simulink model "krzywdalab_tf_si"  (R2023b)
settings: Solver=VariableStepAuto  StartTime=0.0  StopTime=10.0  RelTol=1e-3
values from neighbouring files (symbols this model uses):
  fwe10 = tab_fwe1(it)    [krzywdalab8.m]
  fwe20 = 0.1 * fwe2max    [krzywdalab8.m]
  h10 = (fwe10 + a1 * h20) / a1    [krzywdalab8.m]
  h20 = (fwe10 + fwe20) / a2    [krzywdalab8.m]
  M = [(A1 * A2) (a_1 * A1 + a_2 * A1 + a_1 * A2) a_1*a_2]    [feedback_cascade_transfer_function.m]    (also in krzywdalab8.m = [(A1*A2) (a1*A1+a2*A1+a1*A2) a1*a2])
  N_11 = [A2 (a_1 + a_2)]    [feedback_cascade_transfer_function.m]    (also in krzywdalab8.m = [A2 (a1+a2)])
  N_21 = [a_1]    [feedback_cascade_transfer_function.m]    (also in krzywdalab8.m = [a1])
  N_22 = [A1 a_1]    [feedback_cascade_transfer_function.m]    (also in krzywdalab8.m = [A1 a1])
  T0 = 2    [feedback_cascade_state.m]    (also in feedback_cascade_transfer_function.m; krzywdalab8.m)
settings Model: Creator=igorkrzywda  LastModifiedBy=igorkrzywda

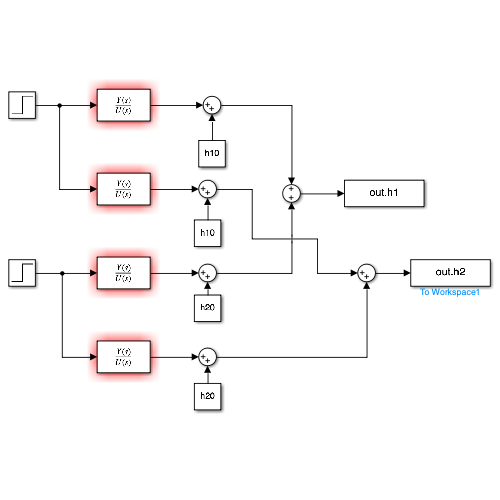
[thumbnail: Simulink's stored preview of the top-level diagram]
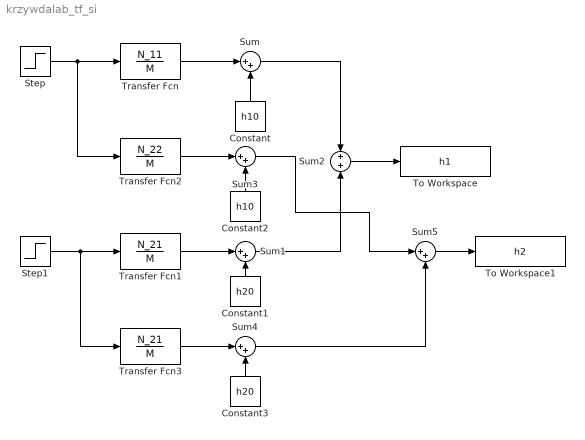
== system krzywdalab_tf_si ==
  Constant : Constant  Value=h10
  Constant1 : Constant  Value=h20
  Constant2 : Constant  Value=h10
  Constant3 : Constant  Value=h20
  Step : Step  Time=T0  After=fwe10  SampleTime=0
  Step1 : Step  Time=T0  After=fwe20  SampleTime=0
  Sum{,1,3..5} (5 alike) : Sum  Inputs=|++
  Sum2 : Sum
  To Workspace : ToWorkspace  VariableName=h1  SampleTime=-1
  To Workspace1 : ToWorkspace  VariableName=h2  SampleTime=-1
  Transfer Fcn : TransferFcn  Numerator=N_11  Denominator=M
  Transfer Fcn1 : TransferFcn  Numerator=N_21  Denominator=M
  Transfer Fcn2 : TransferFcn  Numerator=N_22  Denominator=M
  Transfer Fcn3 : TransferFcn  Numerator=N_21  Denominator=M
  wires:
  Step/1 -> Transfer Fcn2/1, Transfer Fcn/1
  Step1/1 -> Transfer Fcn3/1, Transfer Fcn1/1
  Transfer Fcn/1 -> Sum/1
  Constant/1 -> Sum/2
  Transfer Fcn1/1 -> Sum1/1
  Constant1/1 -> Sum1/2
  Sum/1 -> Sum2/1
  Sum1/1 -> Sum2/2
  Sum2/1 -> To Workspace/1
  Transfer Fcn2/1 -> Sum3/1
  Constant2/1 -> Sum3/2
  Transfer Fcn3/1 -> Sum4/1
  Constant3/1 -> Sum4/2
  Sum3/1 -> Sum5/1
  Sum4/1 -> Sum5/2
  Sum5/1 -> To Workspace1/1
